simulink model "4.3.1"  (R2021a)
settings: Solver=ode3  StartTime=0.0  StopTime=30  FixedStep=0.01  RelTol=1e-3  EnableMultiTasking=on
settings Model: Creator=Oceaner  LastModifiedBy=Oceaner

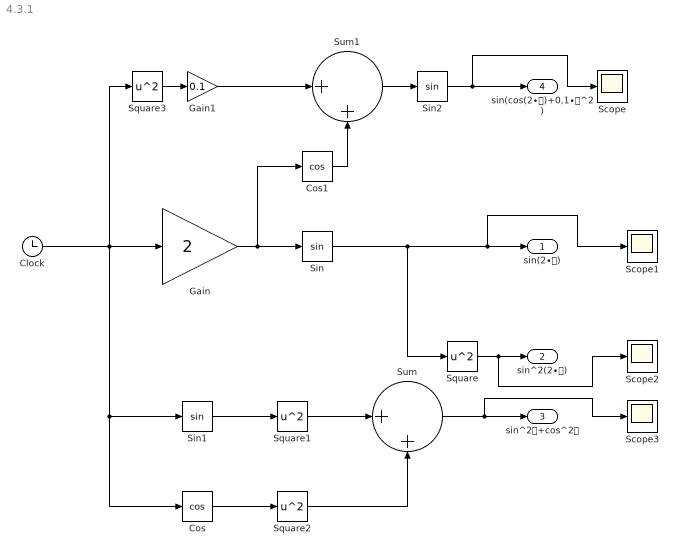
== system 4.3.1 ==
  Clock : Clock
  Cos : Trigonometry  Operator=cos
  Cos1 : Trigonometry  Operator=cos
  Gain : Gain  Gain=2
  Gain1 : Gain  Gain=0.1
  Scope{,1..3} (4 alike) : Scope
  Sin : Trigonometry
  Sin1 : Trigonometry
  Sin2 : Trigonometry
  Square{,1..3} (4 alike) : Math  Operator=square  SaturateOnIntegerOverflow=on
  Sum : Sum  Inputs=|++
  Sum1 : Sum  Inputs=|++
  sin(2∙𝑡) : Outport
  sin^2(2∙𝑡) : Outport  Port=2
  sin^2𝑡+cos^2𝑡 : Outport  Port=3
  sin(cos(2∙𝑡)+0,1∙𝑡^2) : Outport  Port=4
  wires:
  Clock/1 -> Square3/1, Cos/1, Sin1/1, Gain/1
  Gain/1 -> Cos1/1, Sin/1
  Sin/1 -> Square/1, Scope1/1, sin(2∙𝑡)/1
  Square/1 -> Scope2/1, sin^2(2∙𝑡)/1
  Sin1/1 -> Square1/1
  Cos/1 -> Square2/1
  Sum/1 -> Scope3/1, sin^2𝑡+cos^2𝑡/1
  Square1/1 -> Sum/1
  Square2/1 -> Sum/2
  Cos1/1 -> Sum1/2
  Square3/1 -> Gain1/1
  Gain1/1 -> Sum1/1
  Sum1/1 -> Sin2/1
  Sin2/1 -> Scope/1, sin(cos(2∙𝑡)+0,1∙𝑡^2)/1
